simulink model "ex3_p1"  (R2018a)
settings: Solver=VariableStepAuto  StartTime=0.0  StopTime=0.04  MaxStep=1e-6  RelTol=1e-3
libraries: powerlib x8
settings Model: Creator=Administrator  LastModifiedBy=Administrator

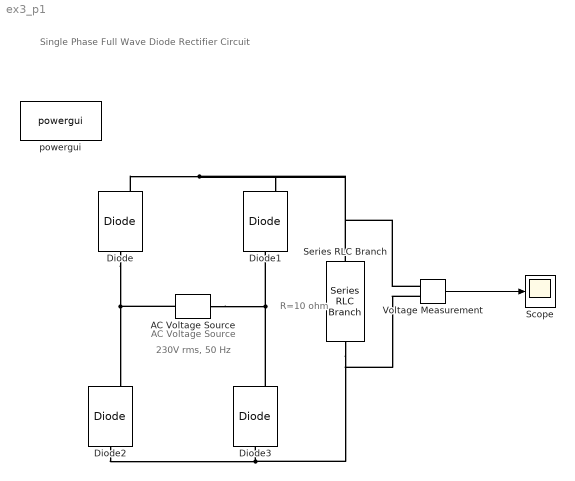
== system ex3_p1 ==
  note: Single Phase Full Wave Diode Rectifier Circuit
  note: 230V rms, 50 Hz
  note: AC Voltage Source
  note: R=10 ohm
  AC Voltage Source : powerlib/Electrical Sources/AC Voltage Source  Amplitude=230  Phase=0  Frequency=50  SampleTime=0  Measurements=None  BusType=swing  Pref=10e3  Qref=0  Qmin=-inf  Qmax=+inf
  Diode{,1..3} (4 alike) : powerlib/Power Electronics/Diode  Ron=0.001  Lon=0  Vf=0.8  IC=0  UseSnubber=0  Rs=500  Cs=250e-9  Measurements=on
  Scope : Scope
  Series RLC Branch : powerlib/Elements/Series RLC Branch  LConnTagsString=__new0  RConnTagsString=__new0  BranchType=R  Resistance=10  Inductance=1e-3  SetiL0=off  InitialCurrent=0  Capacitance=1e-6  Setx0=off  InitialVoltage=0  Measurements=None
  Voltage Measurement : powerlib/Measurements/Voltage Measurement  PhasorSimulation=off  OutputType=Complex  PSBequivalent=0
  powergui : powerlib/powergui  Priority=1  SimulationMode=Continuous  SampleTime=50e-6  frequency=60  Iterations=50  frequencyindice=50  Pbase=100e6  ErrMax=1e-4  UnitsV=kV  UnitsW=MW  buscounter=0  FunctionMessages=off  echomessages=off  EnableUseOfTLC=off  CurrentSourceSwitches=off  DisableSnubberDevices=off  DisableRonSwitches=off  DisableVfSwitches=off  DisplayEquations=off  SolverType=Tustin/Backward Euler (TBE)  Interpol=off  ExternalGateDelay=off  methode=off  Ts=100  x0status=zero  SPID=on  SwTol=0  HookPort=off  RestoreLinks=warning  ResistiveCurrentMeasurement=off  Frange=[0:2:500]  Ylog=off  Xlog=on  ShowGrid=off  save=off  variable=ZData  structure=0  ZoomFFT=off  StartTime=0.0  cycles=1  DisplayStyle=1  fundamental=60  FreqAxis=off  MaxFrequency=1000  frequencyindicesteady=1  RmsSteady=1  display=off
  wires:
  Voltage Measurement/1 -> Scope/1
  connections:
  Diode2/LConn1 -- Voltage Measurement/LConn2 -- Series RLC Branch/RConn1 -- Diode3/LConn1
  Diode/RConn1 -- Voltage Measurement/LConn1 -- Series RLC Branch/LConn1 -- Diode1/RConn1
  Diode3/RConn1 -- AC Voltage Source/RConn1 -- Diode1/LConn1
  Diode/LConn1 -- AC Voltage Source/LConn1 -- Diode2/RConn1
